simulink model "evswitchingblock"  (R2021a)
settings: Solver=VariableStepAuto  StartTime=0.0  StopTime=10.0  RelTol=1e-3
settings Model: Creator=Dell  LastModifiedBy=Dell

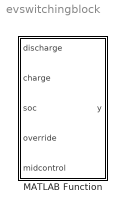
== system evswitchingblock ==
  MATLAB Function : MATLAB Function  TreatAsAtomicUnit=on

== matlab function evswitchingblock/MATLAB Function ==
  data: discharge input; y output; charge input; soc input; override input; midcontrol input
function y = fcn(discharge,charge,soc,override,midcontrol)

if(soc<8.995 && override==0)
    y = charge;
else
    if(soc<8.995 && override==1)
        y = discharge;
    else
        if(soc>9.005 && override==0)
        y = discharge; 
        else
           if(soc>9.005 && override==1)
             y = charge; 
           else
               if(midcontrol == 0)
                   y =charge;
               else
                   y = discharge;
               end
           end
        end
    end
end
